simulink model "irregular_waves"  (R2018b)
settings: Solver=ode4  StartTime=0.0  StopTime=300  FixedStep=0.02  RelTol=1e-3
undefined symbols (not defined in the file or in its folder): heave, SS_discrete, SS_full, SS_inverse, surge
libraries: simulink x1
settings Model: Creator=user  LastModifiedBy=user

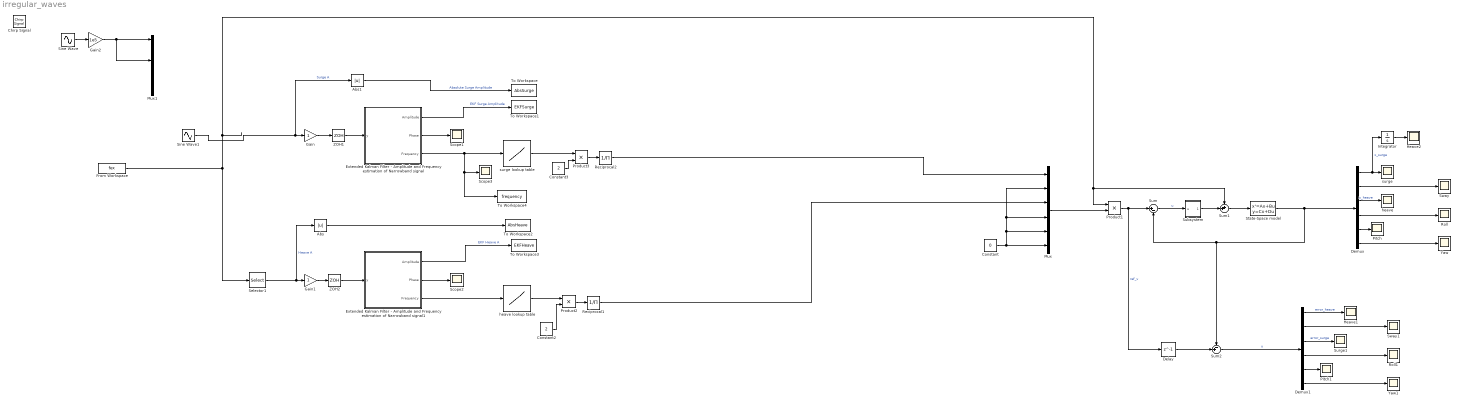
== system irregular_waves ==
  Abs : Abs
  Abs1 : Abs
  Chirp Signal : simulink/Sources/Chirp Signal  f1=0.1  T=100  f2=1
  Constant : Constant  Value=0
  Constant2 : Constant  Value=2
  Constant3 : Constant  Value=2
  Delay : Delay  DelayLength=1  InitialCondition=0
  Demux : Demux  Outputs=6
  Demux1 : Demux  Outputs=6
  Extended Kalman Filter - Amplitude and Frequency estimation of Narrowband signal : MATLAB Function  TreatAsAtomicUnit=on
  Extended Kalman Filter - Amplitude and Frequency estimation of Narrowband signal1 : MATLAB Function  TreatAsAtomicUnit=on
  From Workspace : FromWorkspace  VariableName=fex  SampleTime=0
  Gain : Gain
  Gain1 : Gain
  Gain2 : Gain  Gain=1e5
  Heave1 : Scope
  Heave2 : Scope
  Integrator : Integrator
  Mux : Mux  Inputs=6
  Mux1 : Mux  Inputs=6
  Pitch : Scope
  Pitch1 : Scope
  Product1 : Product
  Product2 : Product
  Product3 : Product
  Reciprocal1 : Product  Inputs=/
  Reciprocal2 : Product  Inputs=/
  Roll : Scope
  Roll1 : Scope
  Scope1 : Scope
  Scope2 : Scope
  Scope3 : Scope
  Selector1 : Selector  InputPortWidth=6  IndexOptions=Index vector (dialog)  Indices=3  OutputSizes=1
  Sine Wave : Sin  Frequency=pi  SampleTime=0
  Sine Wave1 : Sin  Amplitude=10^6  Frequency=0.1  SampleTime=0
  State-Space model : StateSpace  A=SS_full.A  B=SS_full.B  C=SS_full.C  D=SS_full.D  InitialCondition=0
  Subsystem : Subsystem
      mask Display: fprintf("K")
  Sum : Sum  Inputs=|+-
  Sum1 : Sum  Inputs=++|
  Sum2 : Sum  Inputs=-+|
  Surge1 : Scope
  Sway : Scope
  Sway1 : Scope
  To Workspace : ToWorkspace  VariableName=AbsSurge  SaveFormat=Timeseries  SampleTime=-1
  To Workspace1 : ToWorkspace  VariableName=EKFSurge  SaveFormat=Timeseries  SampleTime=-1
  To Workspace2 : ToWorkspace  VariableName=AbsHeave  SaveFormat=Timeseries  SampleTime=-1
  To Workspace3 : ToWorkspace  VariableName=EKFHeave  SaveFormat=Timeseries  SampleTime=-1
  To Workspace4 : ToWorkspace  VariableName=frequency  SaveFormat=Timeseries  SampleTime=-1
  Yaw : Scope
  Yaw1 : Scope
  ZOH1 : ZeroOrderHold  SampleTime=0.02
  ZOH2 : ZeroOrderHold  SampleTime=0.02
  heave : Scope
  heave lookup table : Lookup_n-D  NumberOfTableDimensions=1  BreakpointsForDimension1=heave.freq  Table=heave.amp  InternalRulePriority=Speed  RndMeth=Simplest  InputSameDT=on
  surge : Scope
  surge lookup table : Lookup_n-D  NumberOfTableDimensions=1  BreakpointsForDimension1=surge.freq  Table=surge.amp  InternalRulePriority=Speed  RndMeth=Simplest  InputSameDT=on
  wires:
  Constant/1 -> Mux/2, Mux/4, Mux/5, Mux/6
  Mux/1 -> Product1/2
  Product1/1 -> Delay/1, Sum/1  "ref_v"
  Demux/1 -> Integrator/1, surge/1  "x_surge"
  Demux/3 -> heave/1  "x_heave"
  Demux/5 -> Pitch/1
  Sum1/1 -> State-Space model/1
  Sum/1 -> Subsystem/1(u)  "u"
  Subsystem/1(Out2) -> Sum1/2
  Demux/2 -> Sway/1
  Demux/4 -> Roll/1
  Demux/6 -> Yaw/1
  heave lookup table/1 -> Product2/1
  Constant2/1 -> Product2/2
  Product2/1 -> Reciprocal1/1
  surge lookup table/1 -> Product3/1
  Constant3/1 -> Product3/2
  Product3/1 -> Reciprocal2/1
  Demux1/6 -> Yaw1/1
  Demux1/5 -> Pitch1/1
  Demux1/2 -> Sway1/1
  Demux1/4 -> Roll1/1
  Demux1/3 -> Surge1/1  "error_surge"
  Demux1/1 -> Heave1/1  "error_heave"
  State-Space model/1 -> Demux/1, Sum2/1, Sum/2
  Delay/1 -> Sum2/2
  Sum2/1 -> Demux1/1  "u"
  Extended Kalman Filter - Amplitude and Frequency estimation of Narrowband signal/2(Phase) -> Scope1/1
  Gain/1 -> ZOH1/1
  Sine Wave1/1 -> Abs1/1, Gain/1  "Surge A"
  Extended Kalman Filter - Amplitude and Frequency estimation of Narrowband signal/3(Frequency) -> Scope3/1, To Workspace4/1, surge lookup table/1
  Integrator/1 -> Heave2/1
  From Workspace/1 -> Selector1/1, Product1/1, Sum1/1
  Extended Kalman Filter - Amplitude and Frequency estimation of Narrowband signal1/3(Frequency) -> heave lookup table/1
  ZOH2/1 -> Extended Kalman Filter - Amplitude and Frequency estimation of Narrowband signal1/1(y)
  Selector1/1 -> Abs/1, Gain1/1  "Heave A"
  Gain1/1 -> ZOH2/1
  Extended Kalman Filter - Amplitude and Frequency estimation of Narrowband signal1/2(Phase) -> Scope2/1
  Reciprocal2/1 -> Mux/1
  Reciprocal1/1 -> Mux/3
  Abs/1 -> To Workspace2/1
  Extended Kalman Filter - Amplitude and Frequency estimation of Narrowband signal1/1(Amplitude) -> To Workspace3/1  "EKF Heave A"
  Abs1/1 -> To Workspace/1  "Absolute Surge Amplitude"
  Extended Kalman Filter - Amplitude and Frequency estimation of Narrowband signal/1(Amplitude) -> To Workspace1/1  "EKF Surge Amplitude"
  Sine Wave/1 -> Gain2/1
  ZOH1/1 -> Extended Kalman Filter - Amplitude and Frequency estimation of Narrowband signal/1(y)
  Gain2/1 -> Mux1/3, Mux1/1

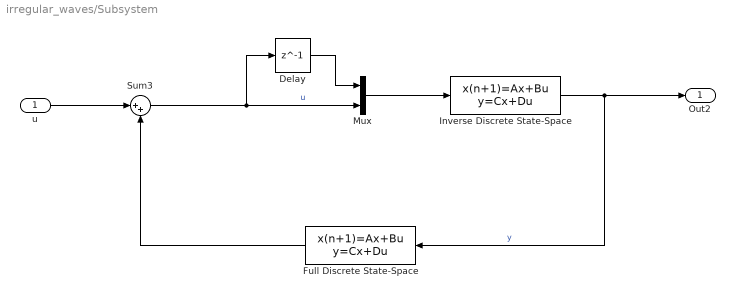
== system irregular_waves/Subsystem ==
  u : Inport
  Delay : Delay  DelayLength=1  InitialCondition=0
  Full Discrete State-Space : DiscreteStateSpace  A=SS_discrete.A  B=SS_discrete.B  C=SS_discrete.C  D=SS_discrete.D  SampleTime=-1
  Inverse Discrete State-Space : DiscreteStateSpace  A=SS_inverse.A  B=SS_inverse.B  C=SS_inverse.C  D=SS_inverse.D  SampleTime=-1
  Mux : Mux  Inputs=2
  Sum3 : Sum  Inputs=|++
  Out2 : Outport
  wires:
  Full Discrete State-Space/1 -> Sum3/2
  Inverse Discrete State-Space/1 -> Full Discrete State-Space/1, Out2/1  "y"
  u/1 -> Sum3/1
  Sum3/1 -> Delay/1, Mux/2  "u"
  Mux/1 -> Inverse Discrete State-Space/1
  Delay/1 -> Mux/1

== matlab function irregular_waves/Extended Kalman Filter - Amplitude and Frequency estimation of Narrowband signal ==
  data: y input; Amplitude output double; Phase output; Frequency output
function [Amplitude, Phase, Frequency]   = EKF_narrowband(y)

% Initialization
persistent P;
persistent x;

dt = 0.02; %edit this to match your timestep

if isempty(P)
    x = [0 0 0.1]';       %state estimate
    P = diag([1e0 1e0 1e0]);    %Covariance matrix
end

%%%%%%%%%%%From Fusco thesis%%%%%%%%%%%%%%%%%%%%%
%%%State vector X = [a theta w]
x1 = x(1);  %Amplitude
x2 = x(2);  %Phase
w = x(3);   %frequency

%State transition matrices
A = [cos(w*dt) sin(w*dt) 0;
    -sin(w*dt) cos(w*dt) 0;
    0 0 1];

q1 = 1e12; q2 = 1e-1; q3 = 1e-1;%Must be comparable to expected magnitudes of each state

% q = [rand*q1 rand*q2 rand*q3]';
% Q = diag(q);
% R=rand*0.1;

q = [q1 q2 q3]';
Q = diag(q);
R=1e-1; %Measurement noise

%Jacobian
dA = [cos(w*dt) sin(w*dt) (-dt*x1*sin(w*dt) + dt*x2*cos(w*dt));
    -sin(w*dt) cos(w*dt) (-dt*x1*cos(w*dt) - dt*x2*sin(w*dt));
     0 0 1];
F = [(x1*cos(w*dt) + x2*sin(w*dt)); (-x1*sin(w*dt) + x2*cos(w*dt)); w];
C = [1 0 0];

%EKF predict/correct
x = A*x;
P = dA*P*dA' + Q;

S = C*P*C' + R;
K = P*C'/S;
x = x + K*(y-C*x);
P = (eye(3) - K*C)*P;

%outputs
Amplitude = sqrt(x(1)^2 + x(2)^2);
Frequency = x(3);
Phase = x(2);

== matlab function irregular_waves/Extended Kalman Filter - Amplitude and Frequency estimation of Narrowband signal1 ==
  data: y input; Amplitude output double; Phase output; Frequency output
function [Amplitude, Phase, Frequency]   = EKF_narrowband(y)

% Initialization
persistent P;
persistent x;

dt = 0.02; %edit this to match your timestep

if isempty(P)
    x = [0 0 0.1]';       %state estimate
    P = diag([1e0 1e0 1e0]);    %Covariance matrix
end

%%%%%%%%%%%From Fusco thesis%%%%%%%%%%%%%%%%%%%%%
%%%State vector X = [a theta w]
x1 = x(1);  %Amplitude
x2 = x(2);  %Phase
w = x(3);   %frequency

%State transition matrices
A = [cos(w*dt) sin(w*dt) 0;
    -sin(w*dt) cos(w*dt) 0;
    0 0 1];

q1 = 1e11; q2 = 1e-1; q3 = 1e-2;%Must be comparable to expected magnitudes of each state

% q = [rand*q1 rand*q2 rand*q3]';
% Q = diag(q);
% R=rand*0.1;

q = [q1 q2 q3]';
Q = diag(q);
R=1e-1; %Measurement noise

%Jacobian
dA = [cos(w*dt) sin(w*dt) (-dt*x1*sin(w*dt) + dt*x2*cos(w*dt));
    -sin(w*dt) cos(w*dt) (-dt*x1*cos(w*dt) - dt*x2*sin(w*dt));
     0 0 1];
F = [(x1*cos(w*dt) + x2*sin(w*dt)); (-x1*sin(w*dt) + x2*cos(w*dt)); w];
C = [1 0 0];

%EKF predict/correct
x = A*x;
P = dA*P*dA' + Q;

S = C*P*C' + R;
K = P*C'/S;
x = x + K*(y-C*x);
P = (eye(3) - K*C)*P;

%outputs
Amplitude = sqrt(x(1)^2 + x(2)^2);
Frequency = x(3);
Phase = x(2);
